simulink model "two_coupled_tanks_turbulent"  (R2020a)
settings: Solver=VariableStepAuto  StartTime=0.0  StopTime=time  RelTol=1e-3
undefined symbols (not defined in the file): qin, resistance1, resistance2, tao1, tao2
settings Model: Creator=jilve  LastModifiedBy=Jilver

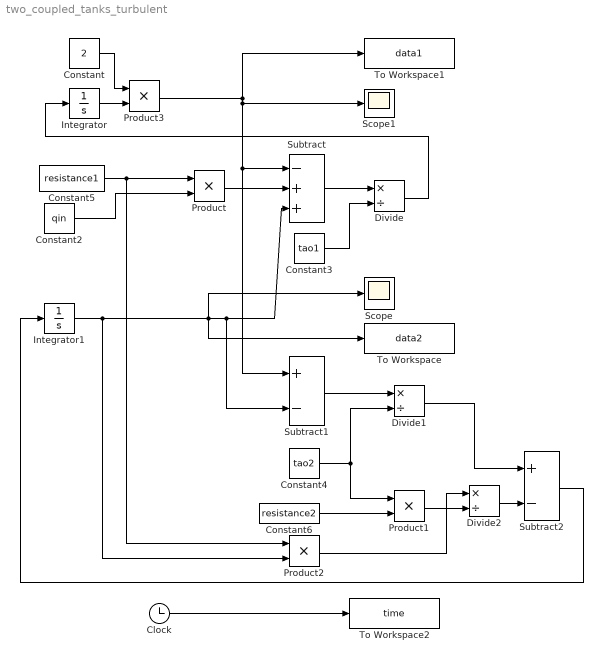
== system two_coupled_tanks_turbulent ==
  Clock : Clock
      settings: Decimation=7000
  Constant : Constant  Value=2
  Constant2 : Constant  Value=qin
  Constant3 : Constant  Value=tao1
  Constant4 : Constant  Value=tao2
  Constant5 : Constant  Value=resistance1
  Constant6 : Constant  Value=resistance2
  Divide : Product  Inputs=*/
  Divide1 : Product  Inputs=*/
  Divide2 : Product  Inputs=*/
  Integrator : Integrator
  Integrator1 : Integrator
  Product{,1..3} (4 alike) : Product
  Scope : Scope
  Scope1 : Scope
  Subtract : Sum  Inputs=-++
  Subtract1 : Sum  Inputs=+-
  Subtract2 : Sum  Inputs=+-
  To Workspace : ToWorkspace  VariableName=data2  SampleTime=-1
  To Workspace1 : ToWorkspace  VariableName=data1  SampleTime=-1
  To Workspace2 : ToWorkspace  VariableName=time  SampleTime=-1
  wires:
  Constant6/1 -> Product1/2
  Constant4/1 -> Product1/1, Divide1/2
  Divide2/1 -> Subtract2/2
  Clock/1 -> To Workspace2/1
  Constant3/1 -> Divide/2
  Product1/1 -> Divide2/2
  Subtract1/1 -> Divide1/1
  Divide1/1 -> Subtract2/1
  Product2/1 -> Divide2/1
  Product3/1 -> To Workspace1/1, Subtract1/1, Subtract/1, Scope1/1
  Integrator1/1 -> Product2/2, Scope/1, To Workspace/1, Subtract1/2, Subtract/3
  Divide/1 -> Integrator/1
  Subtract/1 -> Divide/1
  Subtract2/1 -> Integrator1/1
  Constant2/1 -> Product/2
  Constant5/1 -> Product2/1, Product/1
  Product/1 -> Subtract/2
  Integrator/1 -> Product3/2
  Constant/1 -> Product3/1
